simulink model "mpc_tracking"  (R2020b)
settings: Solver=ode4  StartTime=0.0  StopTime=t_sim  FixedStep=Auto  RelTol=1e-3
values from neighbouring files (symbols this model uses):
  A = [9.5310 195.4713; 0 -5.129]    [main.m]
  A_bar = zeros(n*(Np+1), n)    [main.m]
  B = [-7.6354; 8.0736]    [main.m]
  B_bar = zeros(n*(Np+1), q*Np)    [main.m]
  C = [-1 1]    [main.m]
  C_bar = zeros(p*(Np+1), n)    [main.m]
  D_bar = zeros(p*(Np+1), q*Np)    [main.m]
  dU_bound = repmat(du_bound, Np, 1)    [main.m]
  Np = 20    [main.m]
  q = size(B,2)    [main.m]
  Q_bar = blkdiag(Q_cell{:})    [main.m]
  R_bar = blkdiag(R_cell{:})    [main.m]
  ref = 2    [main.m]
  Ts = 0.01    [main.m]
  U0 = zeros(q*Np, 1)    [main.m]
  U_bound = repmat(u_bound, Np, 1)    [main.m]
  x0 = [0; 0]    [main.m]
  X_bound = repmat(x_bound, Np+1, 1)    [main.m]
undefined symbols (not defined in the file or in its folder): Ad, Bd
settings Model: Creator=vince  LastModifiedBy=vince
settings DataIOCC: ReturnWorkspaceOutputs=off

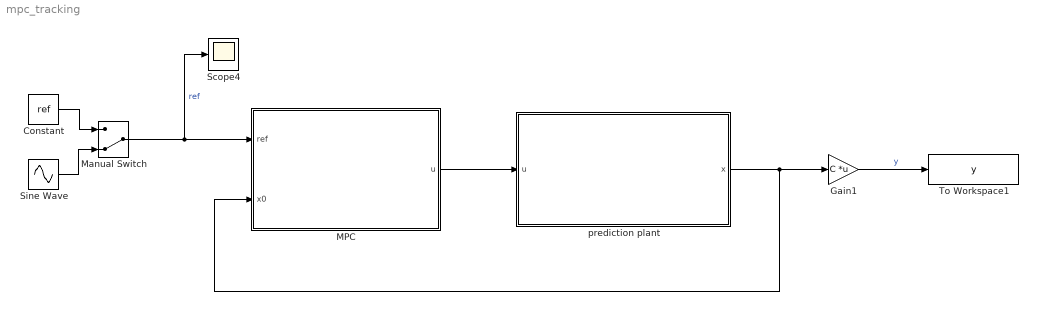
== system mpc_tracking ==
  Constant : Constant  Value=ref  SampleTime=Ts
  Gain1 : Gain  Gain=C  Multiplication=Matrix(K*u) (u vector)
  MPC : Subsystem
  Manual Switch : ManualSwitch  CurrentSetting=0
  Scope4 : Scope
  Sine Wave : Sin  Amplitude=ref  SampleTime=0
  To Workspace1 : ToWorkspace  VariableName=y  SaveFormat=Timeseries  SampleTime=Ts
  prediction plant : Subsystem
  wires:
  Sine Wave/1 -> Manual Switch/2
  Constant/1 -> Manual Switch/1
  Manual Switch/1 -> Scope4/1, MPC/1(ref)  "ref"
  prediction plant/1(x) -> MPC/2(x0), Gain1/1
  MPC/1(u) -> prediction plant/1(u)
  Gain1/1 -> To Workspace1/1  "y"

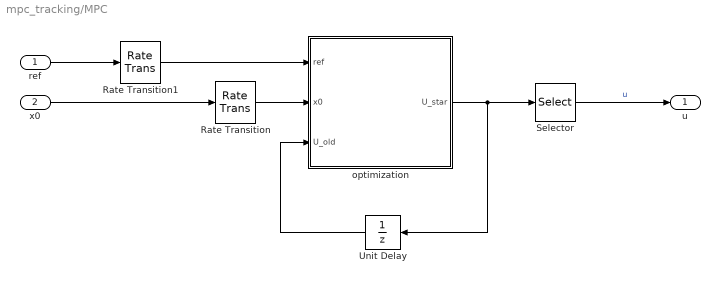
== system mpc_tracking/MPC ==
  ref : Inport
  x0 : Inport  Port=2
  Rate Transition : RateTransition  OutPortSampleTime=Ts
  Rate Transition1 : RateTransition  OutPortSampleTime=Ts
  Selector : Selector  InputPortWidth=q*Np  IndexOptions=Index vector (dialog)  Indices=1:q  OutputSizes=1
  Unit Delay : UnitDelay  InitialCondition=U0  SampleTime=Ts  HasFrameUpgradeWarning=on
  optimization : MATLAB Function  TreatAsAtomicUnit=on
  u : Outport
  wires:
  ref/1 -> Rate Transition1/1
  Unit Delay/1 -> optimization/3(U_old)
  Rate Transition/1 -> optimization/2(x0)
  optimization/1(U_star) -> Unit Delay/1, Selector/1
  Rate Transition1/1 -> optimization/1(ref)
  Selector/1 -> u/1  "u"
  x0/1 -> Rate Transition/1

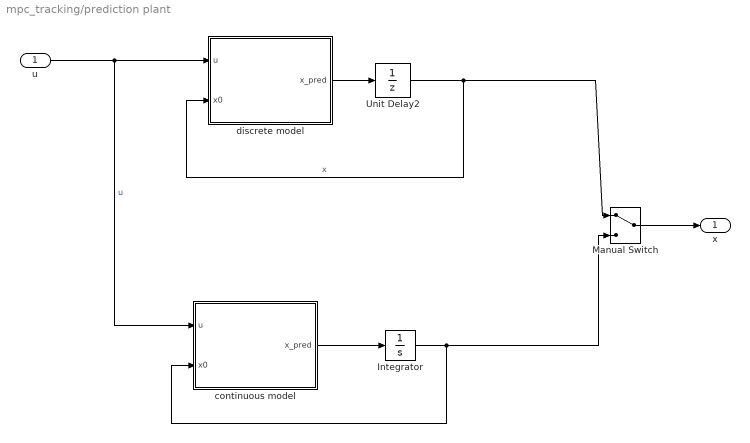
== system mpc_tracking/prediction plant ==
  u : Inport
  Integrator : Integrator  InitialCondition=x0
  Manual Switch : ManualSwitch
  Unit Delay2 : UnitDelay  InitialCondition=x0  SampleTime=Ts  HasFrameUpgradeWarning=on
  continuous model : MATLAB Function  TreatAsAtomicUnit=on
  discrete model : MATLAB Function  TreatAsAtomicUnit=on
  x : Outport
  wires:
  discrete model/1(x_pred) -> Unit Delay2/1
  Unit Delay2/1 -> Manual Switch/1, discrete model/2(x0)  "x"
  continuous model/1(x_pred) -> Integrator/1
  u/1 -> continuous model/1(u), discrete model/1(u)  "u"
  Manual Switch/1 -> x/1
  Integrator/1 -> continuous model/2(x0), Manual Switch/2

== matlab function mpc_tracking/MPC/optimization ==
  data: ref input; U_star output; x0 input; U_old input; q parameter; Np parameter; A_bar parameter; B_bar parameter; C_bar parameter; D_bar parameter; R_bar parameter; Q_bar parameter; X_bound parameter; U_bound parameter; dU_bound parameter
function U_star   = mpc_optimization(ref, x0, U_old, q, Np, A_bar, B_bar, C_bar, D_bar, R_bar, Q_bar, X_bound, U_bound, dU_bound)
%% Documentation
%{
    INCOME: ref, x, U_old
    OUTCOME: U*, X_hat
%}


%% Constraints

REF = repmat(ref, Np+1, 1);


X_min = X_bound(:,1);
X_max = X_bound(:,2);
U_min = U_bound(:,1);
U_max = U_bound(:,2);
dU_min = dU_bound(:,1);
dU_max = dU_bound(:,2);


A_ineq = [-B_bar; B_bar;
        -eye(q*Np); eye(q*Np); 
        -eye(q*Np); eye(q*Np)];
b_ineq = [-X_min+A_bar*x0; X_max-A_bar*x0;
        -U_min; U_max;
        -dU_min-U_old; dU_max+U_old];

    
%% Objective function

H = R_bar + D_bar'*Q_bar*D_bar;
H = (H+H')/2;
f = (C_bar*x0-REF)'*Q_bar*(D_bar);


%% Optimization: J(u(k)) = U(k)'*H*U(k) + f'*U(k)

coder.extrinsic('quadprog');
% options = optimoptions('quadprog', 'Algorithm', 'active-set', 'Display', 'iter');

U_star = zeros(q*Np, 1);
U_star = quadprog(H, f, A_ineq, b_ineq, [], [], [], [], []);

== matlab function mpc_tracking/prediction plant/continuous model ==
  data: u input; x_pred output; x0 input; A parameter; B parameter
function x_pred = mpc_pred_cont(u, x0, A, B)

x = x0;
x_pred = A*x + B*u;

== matlab function mpc_tracking/prediction plant/discrete model ==
  data: u input; x_pred output; x0 input; Ad parameter; Bd parameter
function x_pred = mpc_pred_disc(u, x0, Ad, Bd)

x = x0;
x_pred = Ad*x + Bd*u;
